simulink model "DAQ_DIG_Test"  (Simulink 4.00)
settings: Solver=FixedStepDiscrete  StartTime=0.0  StopTime=inf  FixedStep=0.05  RelTol=1e-3
libraries: DAQ_DIG_lib x1, simulink3 x1
settings Model: LastModifiedBy=bsaunder

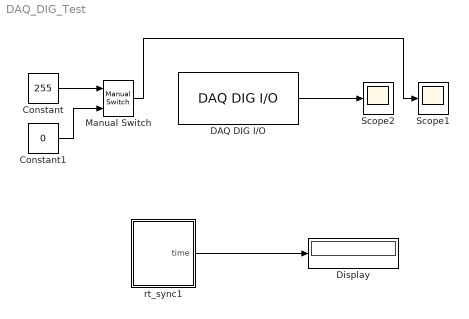
== system DAQ_DIG_Test ==
  Constant : Constant  Value=255
  Constant1 : Constant  Value=0
  DAQ DIG I/O : DAQ_DIG_lib/DAQ DIG I//O  h_mode=no-handshaking (nonlatched)  port_dir=Input (read from DIG port)  port=0  Ts=0.05
  Display : Display
      settings: Format=short
  Manual Switch : simulink3/Nonlinear/Manual Switch  sw=0  action=0
  Scope1 : Scope
      settings: TimeRange=60  YMin=242.25  YMax=267.75  SaveToWorkspace=off  LimitDataPoints=on  MaxDataPoints=5000
  Scope2 : Scope
      settings: TimeRange=60  YMin=0  YMax=275  SaveToWorkspace=off  SaveName=ScopeData  LimitDataPoints=on  MaxDataPoints=5000
  rt_sync1 : Subsystem  mask{Ts=0.05}
      mask prompts: Ts "Sample Time"
      settings: RTWFcnNameOpts=Auto  RTWFileNameOpts=Auto
      mask Display: fprintf('Real\n Time\n sync')
  wires:
  rt_sync1/1(time) -> Display/1
  Constant/1 -> Manual Switch/1
  Constant1/1 -> Manual Switch/2
  Manual Switch/1 -> Scope1/1
  DAQ DIG I/O/1 -> Scope2/1

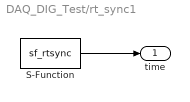
== system DAQ_DIG_Test/rt_sync1 ==
  S-Function : S-Function  FunctionName=sf_rtsync  Parameters=Ts  PortCounts=[]  SFunctionModules=''
  time : Outport  Port=1
  wires:
  S-Function/1 -> time/1
